simulink model "uz_codegen"  (R2025a)
settings: Solver=FixedStepDiscrete  StartTime=0.0  StopTime=50  RelTol=1e-3  EnableMultiTasking=on
PreLoadFcn:
  | uz_setCodegenPaths
model workspace (MATLAB code in the model file):
  | cmdLim = Simulink.Parameter;
  | cmdLim.Value = 15;
  | cmdLim.Description = 'Limit for controlling the maximum surface command angle.';
  | cmdLim.Min = 0;
  | cmdLim.Max = 90;
  | cmdLim.DocUnits = 'deg';
  | 
  | dispGain = Simulink.Parameter;
  | dispGain.Value = 0.75;
  | dispGain.Description = 'Gain applied to the displacement error.';
  | dispGain.Min = 0;
  | dispGain.Max = [];
  | dispGain.DocUnits = 'deg/sec/deg';
  | 
  | dispLim = Simulink.Parameter;
  | dispLim.Value = 30;
  | dispLim.Description = 'Limit for controlling the maximum commanded angle.';
  | dispLim.Min = 0;
  | dispLim.Max = 180;
  | dispLim.DocUnits = 'deg';
  | 
  | intGain = Simulink.Parameter;
  | intGain.Value = 0.5;
  | intGain.Description = 'Gain applied to the integral error.';
  | intGain.Min = 0;
  | intGain.Max = [];
  | intGain.DocUnits = 'deg/sec/deg/sec';
  | 
  | intLim = Simulink.Parameter;
  | intLim.Value = 5;
  | intLim.Description = 'Limit for controlling the maximum commanded angle.';
  | intLim.Min = 0;
  | intLim.Max = 90;
  | intLim.DocUnits = 'deg';
  | 
  | rateGain = Simulink.Parameter;
  | rateGain.Value = 2;
  | rateGain.Description = 'Gain applied to the rate error.';
  | rateGain.Min = 0;
  | rateGain.Max = [];
  | rateGain.DocUnits = 'deg/deg/sec';
  | 
  | rateLim = Simulink.Parameter;
  | rateLim.Value = 6;
  | rateLim.Description = 'Limit for controlling the maximum commanded angle.';
  | rateLim.Min = 0;
  | rateLim.Max = 180;
  | rateLim.DocUnits = 'deg/sec';
  | 
  | hdgGain = Simulink.Parameter;
  | hdgGain.Value = 0.015;
values from neighbouring files (symbols this model uses):
  DIVIDE_ONE_BY_SQRT_THREE = Simulink.Parameter    [PMSMctrl_param.m]
  GAIN_RADS_TO_HZ = Simulink.Parameter    [PMSMctrl_param.m]
  GAIN_UMIN_TO_HZ = Simulink.Parameter    [PMSMctrl_param.m]
  struct_Ctrl_Config = Simulink.Parameter    [config_Ctrl.m]    (also in paramCtrl.m)
  struct_Inv_Config = Simulink.Parameter    [Inverter_Config.m]
  struct_PMSM_Config = Simulink.Parameter    [PMSM_Config.m]
  struct_ZM_In = Simulink.Parameter    [config_Bus_ZM_in.m]
undefined symbols (not defined in the file or in its folder): ctrl_Tsample, mosfet_deadtime, pwr_Udc, Soll_Regelungsart_en
libraries: mySLLib x8, simulink x7, simulink_extras x2
settings Model: RequirementInfo={} %GIDa_fe9045fd_0412_4b6e_8206_617cc20e6fde  FPTRunName=Active  Creator=ts  LastModifiedBy=jonat
settings SolverCC: AlgebraicLoopSolver=TrustRegion  PositivePriorityOrder=on  AutoInsertRateTranBlk=on
settings DataIOCC: SaveOutput=off  SignalLogging=off  DSMLogging=off  SaveTime=off
settings OptimizationCC: DefaultParameterBehavior=Inlined  UseDivisionForNetSlopeComputation=on  GainParamInheritBuiltInType=on  UseFloatMulNetSlope=on  UseSpecifiedMinMax=on  InlineInvariantSignals=on  PassReuseOutputArgsAs=Individual arguments  NoFixptDivByZeroProtection=on  EfficientFloat2IntCast=on  LifeSpan=1  MaxStackSize=64  OptimizeBlockOrder=speed  DifferentSizesBufferReuse=on  EfficientTunableParamExpr=on
settings DebuggingCC: UnconnectedInputMsg=warning  UnconnectedOutputMsg=warning  UnconnectedLineMsg=warning  BusObjectLabelMismatch=error  AllowSymbolicDim=off  SFUnexpectedBacktrackingDiag=warning  SFNoUnconditionalDefaultTransitionDiag=warning  SFExecutionAtInitializationDiag=none  ArithmeticOperatorsInVariantConditions=warning
settings HardwareCC: ProdBitPerPointer=32.0  ProdBitPerSizeT=32.0  ProdBitPerPtrDiffT=32.0  ProdLargestAtomicInteger=Long  ProdLargestAtomicFloat=Double  ProdWordSize=32.0  ProdLongLongMode=on  ProdHWDeviceType=ARM Compatible->ARM Cortex-R  HardwareBoardFeatureSet=SoCBlockset
settings ModelReferenceCC: EnableRefExpFcnMdlSchedulingChecks=on
settings SFSimCC: MATLABDynamicMemAlloc=off
settings RTWCC: SystemTargetFile=ert.tlc  GenCodeOnly=on  TemplateMakefile=ert_default_tmf  GenerateReport=on  BuildConfiguration=Faster Runs  IncludeHyperlinkInReport=on  DataTypeReplacement=CDataTypesFixedWidth  GenerateCodeMetricsReport=on  CheckMdlBeforeBuild=Warning  GPUComputeCapability=3.5  DLArmComputeVersion=19.05  Description=Embedded Coder
settings CodeAppCC: ForceParamTrailComments=on  IgnoreCustomStorageClasses=off  OperatorAnnotations=on  SimulinkDataObjDesc=on  SFDataObjDesc=on  MATLABFcnDesc=on  CustomSymbolStrGlobalVar=rt$N$M  CustomSymbolStrType=$N$M  CustomSymbolStrFcn=$N$M$F  CustomSymbolStrMacro=$N$M  InsertBlockDesc=on  StateflowObjectComments=on  MATLABSourceComments=on  EnableCustomComments=on  ReqsInCode=on
settings ERTTargetCC: ExtModeTransport=0.0  ExtModeStaticAlloc=off  ExtModeMexFile=ext_comm  ExtModeIntrfLevel=Level1  MultiInstanceErrorCode=Warning  RootIOFormat=Part of model data structure  ERTCustomFileTemplate=example_file_process.tlc  GlobalDataDefinition=InSourceFile  GlobalDataReference=InSourceFile  ERTFilePackagingFormat=CompactWithDataFile  MaxIdInt64=INT64_MAX  MinIdInt64=INT64_MIN  MaxIdUint64=UINT64_MAX  MaxIdInt32=INT32_MAX  MinIdInt32=INT32_MIN  MaxIdUint32=UINT32_MAX  MaxIdInt16=INT16_MAX  MinIdInt16=INT16_MIN  MaxIdUint16=UINT16_MAX  MaxIdInt8=INT8_MAX  MinIdInt8=INT8_MIN  MaxIdUint8=UINT8_MAX  DynamicArrayContainerType=coder::array  TargetLangStandard=C99 (ISO)  CodeReplacementLibrary=GNU C99 extensions  MultiwordLength=2048.0  IncludeMdlTerminateFcn=off  CombineSignalStateStructs=on  SuppressErrorStatus=on  IncludeFileDelimiter=UseQuote  SupportAbsoluteTime=off  CodeInterfacePackaging=Reusable function  SupportNonFinite=off  RemoveResetFunc=off  ParenthesesLevel=Minimum
settings ConfigComp: CovScope=ReferencedModels  CovSaveName=covdata_rollAP  CovMetricSettings=dcmtrwe  CovHTMLOptions=-sRT=1 -aTS=1 -bRG=1 -bTC=1 -hTR=1 -nFC=0 -scm=1 -bcm=1 -xEv=0  CovSaveCumulativeToWorkspaceVar=on  CovSaveSingleToWorkspaceVar=on  CovCumulativeVarName=covCumulativeData_rollAP  CovReportOnPause=off  CovExternalEMLEnable=off  CovSFcnEnable=off

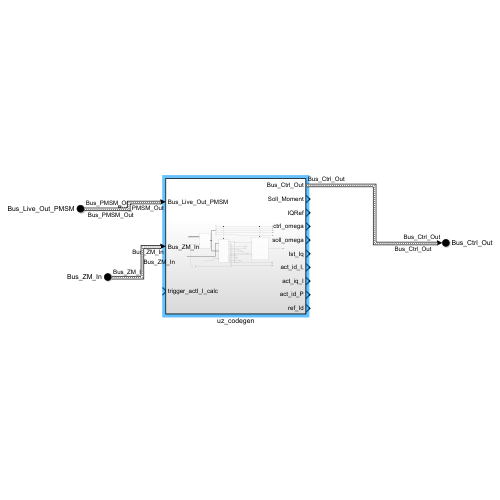
[thumbnail: Simulink's stored preview of the top-level diagram]
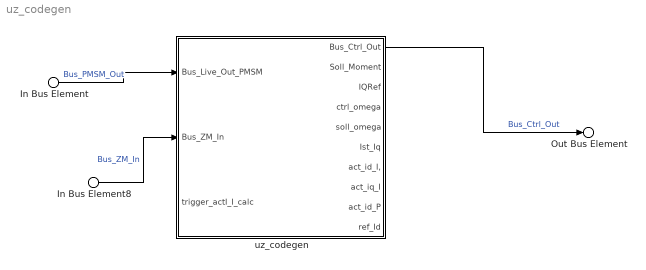
== system uz_codegen ==
  In Bus Element : Inport  PortName=Bus_Live_Out_PMSM
  In Bus Element8 : Inport  Port=2  PortName=Bus_ZM_In
  uz_codegen : Subsystem
  Out Bus Element : Outport  PortName=Bus_Ctrl_Out
  wires:
  In Bus Element8/1 -> uz_codegen/2(Bus_ZM_In)  "Bus_ZM_In"
  In Bus Element/1 -> uz_codegen/1(Bus_Live_Out_PMSM)  "Bus_PMSM_Out"
  uz_codegen/1(Bus_Ctrl_Out) -> Out Bus Element/1  "Bus_Ctrl_Out"

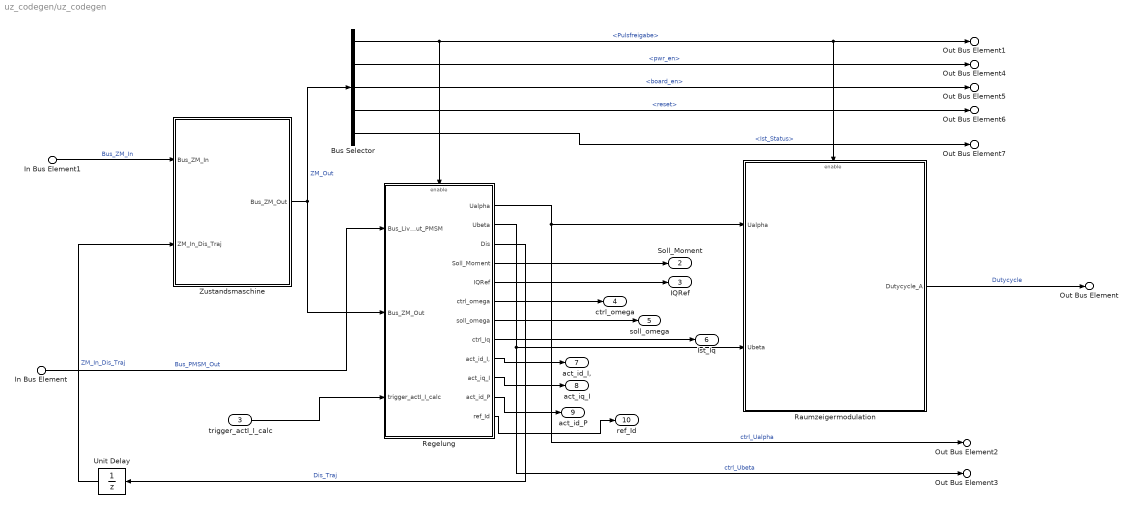
== system uz_codegen/uz_codegen ==
  In Bus Element : Inport  PortName=Bus_Live_Out_PMSM
  In Bus Element1 : Inport  Port=2  PortName=Bus_ZM_In
  trigger_actI_I_calc : Inport  Port=3
  Bus Selector : BusSelector  OutputSignals=Pulsfreigabe,pwr_en,board_en,reset,Ist_Status
  Raumzeigermodulation : Subsystem  TreatAsAtomicUnit=on
      settings: RTWFcnNameOpts=Use subsystem name
  Regelung : Subsystem
      settings: RTWFcnNameOpts=Use subsystem name
  Unit Delay : UnitDelay  SampleTime=-1  HasFrameUpgradeWarning=on
  Zustandsmaschine : Subsystem  TreatAsAtomicUnit=on
      settings: RTWFcnNameOpts=Use subsystem name
  Out Bus Element : Outport  PortName=Bus_Ctrl_Out  Element=Dutycycle
  Out Bus Element1 : Outport  PortName=Bus_Ctrl_Out  Element=act_pwm
  Out Bus Element2 : Outport  PortName=Bus_Ctrl_Out  Element=ctrl_Ualpha_V
  Out Bus Element3 : Outport  PortName=Bus_Ctrl_Out  Element=ctrl_Ubeta_V
  Out Bus Element4 : Outport  PortName=Bus_Ctrl_Out  Element=pwr_en
  Out Bus Element5 : Outport  PortName=Bus_Ctrl_Out  Element=board_en
  Out Bus Element6 : Outport  PortName=Bus_Ctrl_Out  Element=reset
  Out Bus Element7 : Outport  PortName=Bus_Ctrl_Out  Element=ZM_Ist_Status
  Soll_Moment : Outport  Port=2
  IQRef : Outport  Port=3
  ctrl_omega : Outport  Port=4
  soll_omega : Outport  Port=5
  Ist_Iq : Outport  Port=6
  act_id_I, : Outport  Port=7
  act_iq_I : Outport  Port=8
  act_id_P : Outport  Port=9
  ref_Id : Outport  Port=10
  wires:
  Bus Selector/3 -> Out Bus Element5/1  "<board_en>"
  Regelung/3(Dis) -> Unit Delay/1  "Dis_Traj"
  Regelung/1(Ualpha) -> Out Bus Element2/1, Raumzeigermodulation/1(Ualpha)  "ctrl_Ualpha"
  Regelung/2(Ubeta) -> Out Bus Element3/1, Raumzeigermodulation/2(Ubeta)  "ctrl_Ubeta"
  Zustandsmaschine/1(Bus_ZM_Out) -> Regelung/2(Bus_ZM_Out), Bus Selector/1  "ZM_Out"
  Bus Selector/4 -> Out Bus Element6/1  "<reset>"
  Unit Delay/1 -> Zustandsmaschine/2(ZM_In_Dis_Traj)  "ZM_In_Dis_Traj"
  In Bus Element1/1 -> Zustandsmaschine/1(Bus_ZM_In)  "Bus_ZM_In"
  Raumzeigermodulation/1(Dutycycle_A) -> Out Bus Element/1  "Dutycycle"
  Bus Selector/1 -> Regelung/Enable, Raumzeigermodulation/Enable, Out Bus Element1/1  "<Pulsfreigabe>"
  Bus Selector/5 -> Out Bus Element7/1  "<Ist_Status>"
  In Bus Element/1 -> Regelung/1(Bus_Live_Out_PMSM)  "Bus_PMSM_Out"
  Bus Selector/2 -> Out Bus Element4/1  "<pwr_en>"
  Regelung/4(Soll_Moment) -> Soll_Moment/1
  Regelung/5(IQRef) -> IQRef/1
  Regelung/6(ctrl_omega) -> ctrl_omega/1
  Regelung/7(soll_omega) -> soll_omega/1
  Regelung/8(ctrl_Iq) -> Ist_Iq/1
  Regelung/9(act_id_I,) -> act_id_I,/1
  Regelung/10(act_iq_I) -> act_iq_I/1
  Regelung/11(act_id_P) -> act_id_P/1
  Regelung/12(ref_Id) -> ref_Id/1
  trigger_actI_I_calc/1 -> Regelung/3(trigger_actI_I_calc)

== system uz_codegen/uz_codegen/Raumzeigermodulation ==
  Ualpha : Inport
  Ubeta : Inport  Port=2
  Enable : EnablePort
  Constant : Constant  Value=struct_Inv_Config.Udc
  MinimaleSchaltzeit : Subsystem
      settings: RTWFcnNameOpts=Use subsystem name
  Mux : Mux  Inputs=3
  Terminator : Terminator
  Terminator1 : Terminator
  raumzeigermodulation : MATLAB Function  TreatAsAtomicUnit=on
      settings: RTWFcnNameOpts=Use subsystem name
  Dutycycle_A : Outport
  wires:
  MinimaleSchaltzeit/1(Out1) -> Dutycycle_A/1
  Mux/1 -> MinimaleSchaltzeit/1(Dutycycle)
  Ubeta/1 -> raumzeigermodulation/2(Ubeta)  "ctrl_Ubeta"
  Ualpha/1 -> raumzeigermodulation/1(Ualpha)  "ctrl_Ualpha"
  raumzeigermodulation/1(Dutycycle_A) -> Mux/1
  raumzeigermodulation/2(Dutycycle_B) -> Mux/2
  raumzeigermodulation/3(Dutycycle_C) -> Mux/3
  Constant/1 -> raumzeigermodulation/3(Udc)
  raumzeigermodulation/4(Sektor) -> Terminator1/1  "Sektor"
  raumzeigermodulation/5(Quadrant) -> Terminator/1

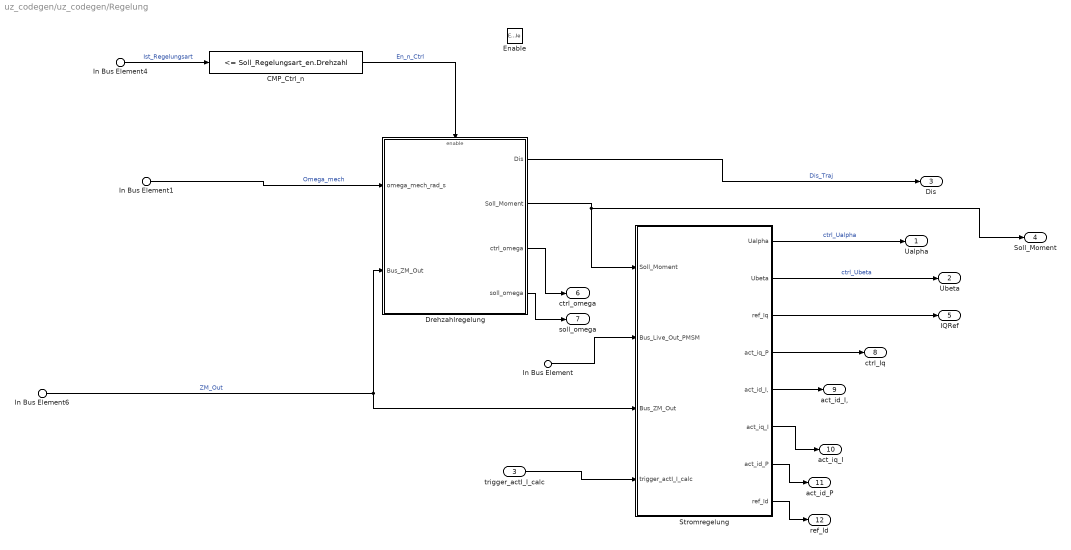
== system uz_codegen/uz_codegen/Regelung ==
  In Bus Element : Inport  PortName=Bus_Live_Out_PMSM
  In Bus Element1 : Inport  PortName=Bus_Live_Out_PMSM  Element=pmsm_Omega_mech_rad_s
  In Bus Element6 : Inport  Port=2  PortName=Bus_ZM_Out
  In Bus Element4 : Inport  Port=2  PortName=Bus_ZM_Out  Element=Ist_Regelungsart
  trigger_actI_I_calc : Inport  Port=3
  Enable : EnablePort  StatesWhenEnabling=reset
  CMP_Ctrl_n : simulink/Logic and Bit Operations/Compare To Constant  relop=<=  const=Soll_Regelungsart_en.Drehzahl  OutDataTypeStr=boolean
  Drehzahlregelung : Subsystem
      settings: RTWFcnNameOpts=Use subsystem name
  Stromregelung : Subsystem  TreatAsAtomicUnit=on
      settings: RTWFcnNameOpts=Use subsystem name
  Ualpha : Outport
  Ubeta : Outport  Port=2
  Dis : Outport  Port=3  OutDataTypeStr=boolean
  Soll_Moment : Outport  Port=4
  IQRef : Outport  Port=5
  ctrl_omega : Outport  Port=6
  soll_omega : Outport  Port=7
  ctrl_Iq : Outport  Port=8
  act_id_I, : Outport  Port=9
  act_iq_I : Outport  Port=10
  act_id_P : Outport  Port=11
  ref_Id : Outport  Port=12
  wires:
  CMP_Ctrl_n/1 -> Drehzahlregelung/Enable  "En_n_Ctrl"
  Drehzahlregelung/2(Soll_Moment) -> Stromregelung/1(Soll_Moment), Soll_Moment/1
  Drehzahlregelung/1(Dis) -> Dis/1  "Dis_Traj"
  In Bus Element1/1 -> Drehzahlregelung/1(omega_mech_rad_s)  "Omega_mech"
  In Bus Element4/1 -> CMP_Ctrl_n/1  "Ist_Regelungsart"
  In Bus Element6/1 -> Drehzahlregelung/2(Bus_ZM_Out), Stromregelung/3(Bus_ZM_Out)  "ZM_Out"
  Stromregelung/2(Ubeta) -> Ubeta/1  "ctrl_Ubeta"
  Stromregelung/1(Ualpha) -> Ualpha/1  "ctrl_Ualpha"
  In Bus Element/1 -> Stromregelung/2(Bus_Live_Out_PMSM)
  Stromregelung/3(ref_Iq) -> IQRef/1
  Drehzahlregelung/3(ctrl_omega) -> ctrl_omega/1
  Drehzahlregelung/4(soll_omega) -> soll_omega/1
  Stromregelung/4(act_iq_P) -> ctrl_Iq/1
  Stromregelung/5(act_id_I,) -> act_id_I,/1
  Stromregelung/6(act_iq_I) -> act_iq_I/1
  Stromregelung/7(act_id_P) -> act_id_P/1
  Stromregelung/8(ref_Id) -> ref_Id/1
  trigger_actI_I_calc/1 -> Stromregelung/4(trigger_actI_I_calc)

== system uz_codegen/uz_codegen/Zustandsmaschine ==
  In Bus Element1 : Inport  PortName=Bus_ZM_In
  ZM_In_Dis_Traj : Inport  Port=2
  state_chart : Stateflow chart  TreatAsAtomicUnit=on
      settings: RTWSystemCode=Nonreusable function  RTWFcnNameOpts=Use subsystem name  FunctionInterfaceSpec=Allow arguments (Optimized)
  Out Bus Element : Outport  PortName=Bus_ZM_Out
  wires:
  ZM_In_Dis_Traj/1 -> state_chart/2(Dis)  "Dis_Traj"
  In Bus Element1/1 -> state_chart/1(Bus_ZM_In)  "Bus_ZM_In"
  state_chart/1(Bus_ZM_Out) -> Out Bus Element/1  "ZM_Out"

== system uz_codegen/uz_codegen/Raumzeigermodulation/MinimaleSchaltzeit ==
  Dutycycle : Inport
  Constant : Constant  Value=struct_Ctrl_Config.IGBT_dc_min
  Constant1 : Constant  Value=0  OutDataTypeStr=single
  Constant2 : Constant  Value=1-struct_Ctrl_Config.IGBT_dc_min
  Constant3 : Constant  OutDataTypeStr=single
  Switch1 : Switch  Threshold=struct_Ctrl_Config.IGBT_dc_min  OutDataTypeStr=single  SaturateOnIntegerOverflow=off  InputSameDT=off
  Switch2 : Switch  Threshold=struct_Ctrl_Config.IGBT_dc_min/2  OutDataTypeStr=single  SaturateOnIntegerOverflow=off  InputSameDT=off
  Switch3 : Switch  Criteria=u2 > Threshold  Threshold=1-struct_Ctrl_Config.IGBT_dc_min  OutDataTypeStr=single  SaturateOnIntegerOverflow=off  InputSameDT=off
  Switch4 : Switch  Threshold=1-struct_Ctrl_Config.IGBT_dc_min/2  OutDataTypeStr=single  SaturateOnIntegerOverflow=off
  Out1 : Outport
  wires:
  Constant/1 -> Switch2/1
  Constant2/1 -> Switch4/3
  Switch3/1 -> Out1/1
  Switch2/1 -> Switch1/3
  Constant3/1 -> Switch4/1
  Dutycycle/1 -> Switch1/2, Switch1/1, Switch2/2
  Switch1/1 -> Switch3/3, Switch3/2, Switch4/2
  Constant1/1 -> Switch2/3
  Switch4/1 -> Switch3/1

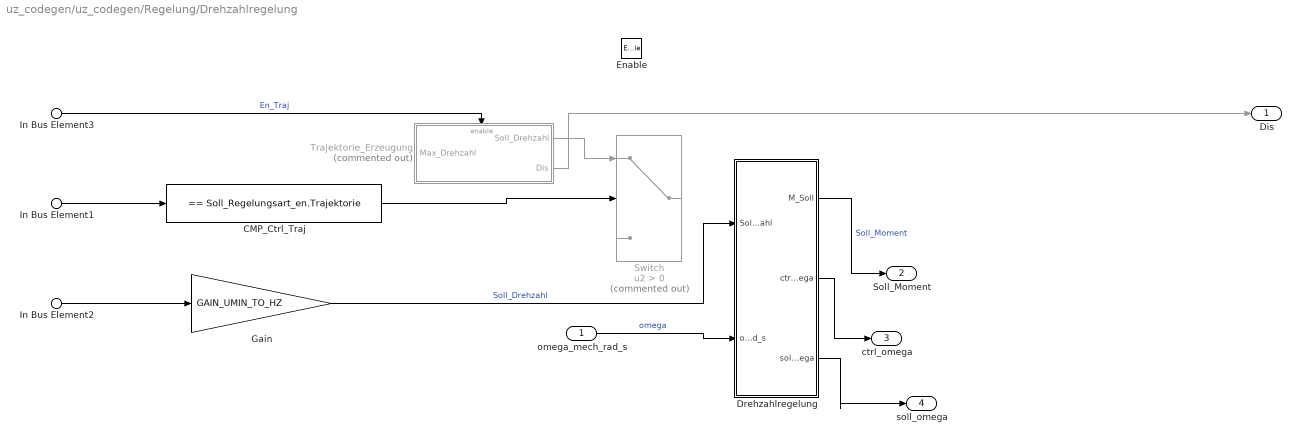
== system uz_codegen/uz_codegen/Regelung/Drehzahlregelung ==
  omega_mech_rad_s : Inport
  In Bus Element3 : Inport  Port=2  PortName=Bus_ZM_Out  Element=En_Traj
  In Bus Element1 : Inport  Port=2  PortName=Bus_ZM_Out  Element=Ist_Regelungsart
  In Bus Element2 : Inport  Port=2  PortName=Bus_ZM_Out  Element=Soll_Drehzahl_Umin
  Enable : EnablePort  StatesWhenEnabling=reset
  CMP_Ctrl_Traj : simulink/Logic and Bit Operations/Compare To Constant  relop===  const=Soll_Regelungsart_en.Trajektorie  OutDataTypeStr=boolean
  Drehzahlregelung : Subsystem
      settings: RTWSystemCode=Nonreusable function  RTWFcnNameOpts=Use subsystem name
  Gain : Gain  Gain=GAIN_UMIN_TO_HZ  RndMeth=Zero
  Switch : Switch  Commented=on  Criteria=u2 > Threshold  SaturateOnIntegerOverflow=off  InputSameDT=off
  Trajektorie_Erzeugung : Subsystem  Commented=on
      settings: RTWSystemCode=Nonreusable function  RTWFcnNameOpts=Use subsystem name
  Dis : Outport
  Soll_Moment : Outport  Port=2
  ctrl_omega : Outport  Port=3
  soll_omega : Outport  Port=4
  wires:
  omega_mech_rad_s/1 -> Drehzahlregelung/2(omega_mech_rad_s)  "omega"
  In Bus Element3/1 -> Trajektorie_Erzeugung/Enable  "En_Traj"
  CMP_Ctrl_Traj/1 -> Switch/2
  In Bus Element1/1 -> CMP_Ctrl_Traj/1
  In Bus Element2/1 -> Gain/1
  Trajektorie_Erzeugung/2(Dis) -> Dis/1
  Gain/1 -> Drehzahlregelung/1(Soll_Drehzahl)  "Soll_Drehzahl"
  Drehzahlregelung/1(M_Soll) -> Soll_Moment/1  "Soll_Moment"
  Trajektorie_Erzeugung/1(Soll_Drehzahl) -> Switch/1
  Drehzahlregelung/2(ctrl_omega) -> ctrl_omega/1
  Drehzahlregelung/3(soll_omega) -> soll_omega/1

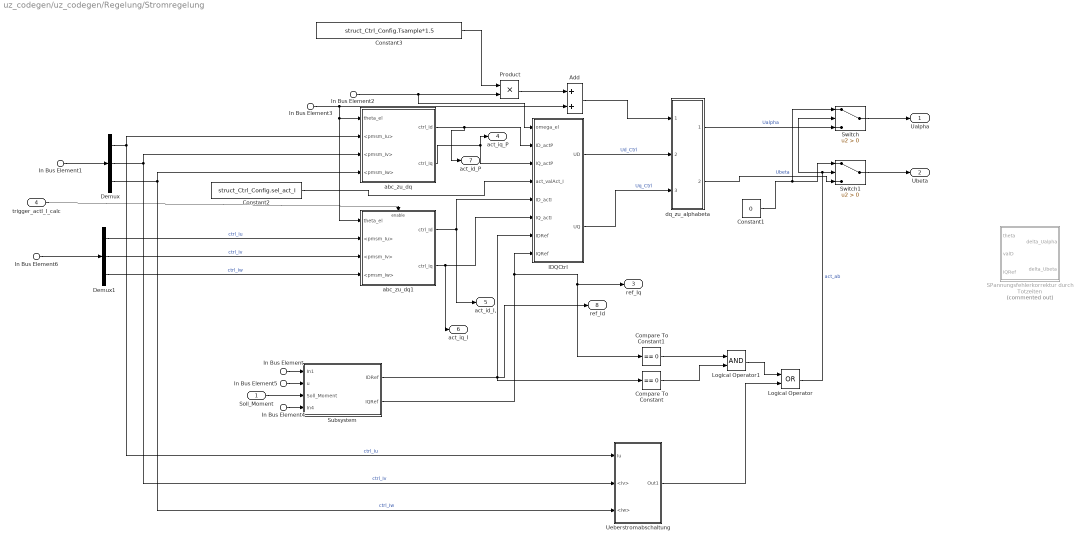
== system uz_codegen/uz_codegen/Regelung/Stromregelung ==
  Soll_Moment : Inport
  In Bus Element1 : Inport  Port=2  PortName=Bus_Live_Out_PMSM  Element=pmsm_Iuvw_P_A
  In Bus Element6 : Inport  Port=2  PortName=Bus_Live_Out_PMSM  Element=pmsm_Iuvw_I_A
  In Bus Element2 : Inport  Port=2  PortName=Bus_Live_Out_PMSM  Element=pmsm_Omega_el_rad_s
  In Bus Element3 : Inport  Port=2  PortName=Bus_Live_Out_PMSM  Element=pmsm_theta_el_rad
  In Bus Element5 : Inport  Port=3  PortName=Bus_ZM_Out  Element=Ist_Regelungsart
  In Bus Element : Inport  Port=3  PortName=Bus_ZM_Out  Element=Soll_id_A
  In Bus Element4 : Inport  Port=3  PortName=Bus_ZM_Out  Element=Soll_iq_A
  trigger_actI_I_calc : Inport  Port=4  OutDataTypeStr=boolean
  Add : Sum
  Compare To Constant : simulink/Logic and Bit Operations/Compare To Constant  relop===  const=0  OutDataTypeStr=boolean
  Compare To Constant1 : simulink/Logic and Bit Operations/Compare To Constant  relop===  const=0  OutDataTypeStr=boolean
  Constant1 : Constant  Value=0  OutDataTypeStr=single
  Constant2 : Constant  Value=struct_Ctrl_Config.sel_act_I  OutDataTypeStr=boolean
  Constant3 : Constant  Value=struct_Ctrl_Config.Tsample*1.5  OutDataTypeStr=single
  Demux : Demux  Outputs=3
  Demux1 : Demux  Outputs=3
  IDQCtrl : Subsystem
      settings: RTWSystemCode=Nonreusable function  RTWFcnNameOpts=Use subsystem name
  Logical Operator : Logic  Operator=OR  AllPortsSameDT=off  OutDataTypeStr=boolean
  Logical Operator1 : Logic  AllPortsSameDT=off  OutDataTypeStr=boolean
  Product : Product
  SPannungsfehlerkorrektur durch Totzeiten : Subsystem  Commented=on
  Subsystem : Subsystem
  Switch : Switch  Criteria=u2 > Threshold  SaturateOnIntegerOverflow=off  InputSameDT=off
  Switch1 : Switch  Criteria=u2 > Threshold  SaturateOnIntegerOverflow=off  InputSameDT=off
  Ueberstromabschaltung : Subsystem
      settings: RTWSystemCode=Nonreusable function  RTWFcnNameOpts=Use subsystem name
  abc_zu_dq : Subsystem
      settings: RTWFcnNameOpts=Use subsystem name
  abc_zu_dq1 : Subsystem
      settings: RTWFcnNameOpts=Use subsystem name
  dq_zu_alphabeta : Subsystem  AncestorBlock=mySLLib/Inverse Park-Transformation
      settings: RTWFcnNameOpts=Use subsystem name
  Ualpha : Outport
  Ubeta : Outport  Port=2
  ref_Iq : Outport  Port=3
  act_iq_P : Outport  Port=4
  act_id_I, : Outport  Port=5
  act_iq_I : Outport  Port=6
  act_id_P : Outport  Port=7
  ref_Id : Outport  Port=8
  wires:
  Logical Operator1/1 -> Logical Operator/1
  Constant3/1 -> Product/1
  In Bus Element1/1 -> Demux/1
  Compare To Constant1/1 -> Logical Operator1/1
  abc_zu_dq/2(ctrl_Iq) -> act_iq_P/1, IDQCtrl/3(IQ_actP)
  abc_zu_dq/1(ctrl_Id) -> act_id_P/1, IDQCtrl/2(ID_actP)
  Compare To Constant/1 -> Logical Operator1/2
  Ueberstromabschaltung/1(Out1) -> Logical Operator/2
  Logical Operator/1 -> Switch/2, Switch1/2  "act_ab"
  Constant1/1 -> Switch/1, Switch1/1
  Switch/1 -> Ualpha/1
  Switch1/1 -> Ubeta/1
  dq_zu_alphabeta/1(valAlpha) -> Switch/3  "Ualpha"
  dq_zu_alphabeta/2(valBeta) -> Switch1/3  "Ubeta"
  IDQCtrl/2(UQ) -> dq_zu_alphabeta/3(valQ)  "Uq_Ctrl"
  Add/1 -> dq_zu_alphabeta/1(theta_el)
  Product/1 -> Add/1
  Demux/1 -> abc_zu_dq/2(<pmsm_Iu>), Ueberstromabschaltung/1(Iu)  "ctrl_Iu"
  Demux/2 -> abc_zu_dq/3(<pmsm_Iv>), Ueberstromabschaltung/2(<Iv>)  "ctrl_Iv"
  In Bus Element3/1 -> abc_zu_dq/1(theta_el), abc_zu_dq1/1(theta_el), Add/2
  Demux/3 -> abc_zu_dq/4(<pmsm_Iw>), Ueberstromabschaltung/3(<Iw>)  "ctrl_Iw"
  In Bus Element2/1 -> IDQCtrl/1(omega_el), Product/2
  IDQCtrl/1(UD) -> dq_zu_alphabeta/2(valD)  "Ud_Ctrl"
  Constant2/1 -> IDQCtrl/4(act_valAct_I)
  Subsystem/1(IDRef) -> ref_Id/1, IDQCtrl/7(IDRef), Compare To Constant/1
  Subsystem/2(IQRef) -> IDQCtrl/8(IQRef), Compare To Constant1/1, ref_Iq/1
  In Bus Element/1 -> Subsystem/1(In1)
  In Bus Element5/1 -> Subsystem/2(u)
  Soll_Moment/1 -> Subsystem/3(Soll_Moment)
  In Bus Element4/1 -> Subsystem/4(In4)
  abc_zu_dq1/1(ctrl_Id) -> IDQCtrl/5(ID_actI), act_id_I,/1
  abc_zu_dq1/2(ctrl_Iq) -> act_iq_I/1, IDQCtrl/6(IQ_actI)
  Demux1/1 -> abc_zu_dq1/2(<pmsm_Iu>)  "ctrl_Iu"
  Demux1/2 -> abc_zu_dq1/3(<pmsm_Iv>)  "ctrl_Iv"
  Demux1/3 -> abc_zu_dq1/4(<pmsm_Iw>)  "ctrl_Iw"
  In Bus Element6/1 -> Demux1/1
  trigger_actI_I_calc/1 -> abc_zu_dq1/Enable

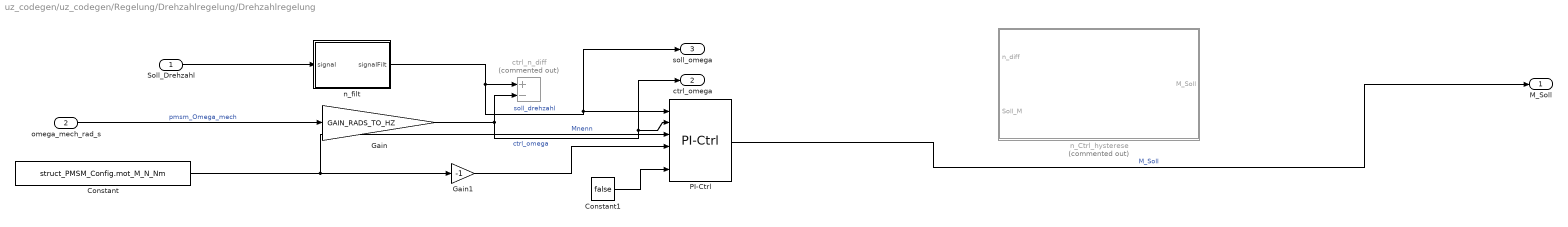
== system uz_codegen/uz_codegen/Regelung/Drehzahlregelung/Drehzahlregelung ==
  Soll_Drehzahl : Inport  OutDataTypeStr=single
  omega_mech_rad_s : Inport  Port=2
  Constant : Constant  Value=struct_PMSM_Config.mot_M_N_Nm  SampleTime=-1
  Constant1 : Constant  Value=false  OutDataTypeStr=boolean
  Gain : Gain  Gain=GAIN_RADS_TO_HZ  OutDataTypeStr=single  RndMeth=Zero
  Gain1 : Gain  Gain=-1
  PI-Ctrl : mySLLib/PI-Ctrl  localGain=struct_Ctrl_Config.KPn  localTsample=struct_Ctrl_Config.Tsample  localKi=struct_Ctrl_Config.KIn
      settings: SourceProductName=MSSS Bibliothek
  ctrl_n_diff : Sum  Commented=on  Inputs=+-
  n_Ctrl_hysterese : Subsystem  Commented=on  TreatAsAtomicUnit=on
  n_filt : Subsystem  AncestorBlock=libKollege/low pass filter  mask{localTFilt=struct_Ctrl_Config.TNn, localTsample=struct_Ctrl_Config.Tsample}
      mask prompts: localTFilt "Filterzeitkonstante (s)"; localTsample "Abtastzeit (s)"
      mask init:
      | if localTsample <= 0
      |     error('Abtastzeit darf nicht kleiner gleich Null sein!')
      | end
      | 
      | if localTFilt <= 0
      |     error('Filterzeit darf nicht kleiner gleich Null sein!')
      | end
  M_Soll : Outport  OutDataTypeStr=single
  ctrl_omega : Outport  Port=2
  soll_omega : Outport  Port=3
  wires:
  Gain1/1 -> PI-Ctrl/4
  Soll_Drehzahl/1 -> n_filt/1(signal)
  omega_mech_rad_s/1 -> Gain/1  "pmsm_Omega_mech"
  Constant/1 -> Gain1/1, PI-Ctrl/3  "Mnenn"
  Gain/1 -> ctrl_omega/1, PI-Ctrl/2, ctrl_n_diff/2  "ctrl_omega"
  n_filt/1(signalFilt) -> ctrl_n_diff/1, soll_omega/1, PI-Ctrl/1  "soll_drehzahl"
  PI-Ctrl/1 -> M_Soll/1  "M_Soll"
  Constant1/1 -> PI-Ctrl/6

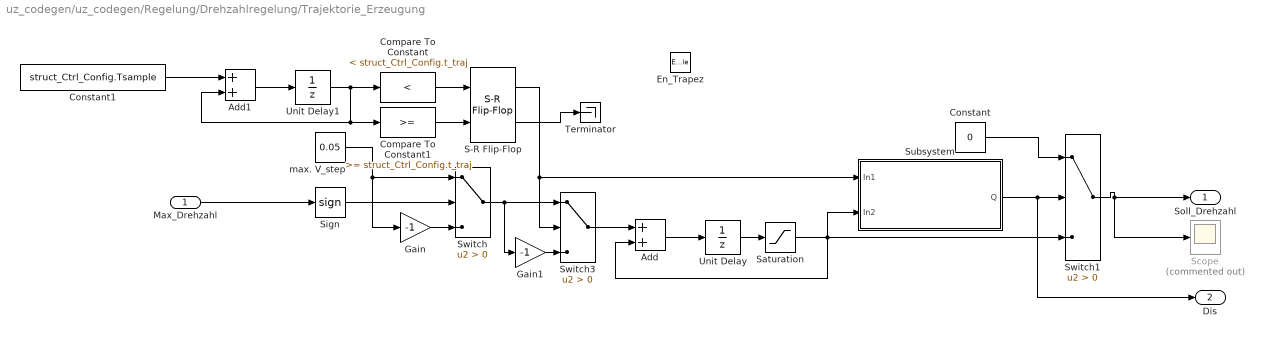
== system uz_codegen/uz_codegen/Regelung/Drehzahlregelung/Trajektorie_Erzeugung ==
  Max_Drehzahl : Inport  OutDataTypeStr=single
  En_Trapez : EnablePort  StatesWhenEnabling=reset
  Add : Sum  OutDataTypeStr=single
  Add1 : Sum  OutDataTypeStr=single
  Compare To Constant : simulink/Logic and Bit Operations/Compare To Constant  relop=<  const=struct_Ctrl_Config.t_traj  OutDataTypeStr=boolean
  Compare To Constant1 : simulink/Logic and Bit Operations/Compare To Constant  relop=>=  const=struct_Ctrl_Config.t_traj  OutDataTypeStr=boolean
  Constant : Constant  Value=0  OutDataTypeStr=single
  Constant1 : Constant  Value=struct_Ctrl_Config.Tsample
  Gain : Gain  Gain=-1
  Gain1 : Gain  Gain=-1
  S-R Flip-Flop : simulink_extras/Flip Flops/S-R Flip-Flop  initial_condition=1
  Saturation : Saturate  UpperLimit=abs(struct_ZM_In.Soll_Drehzahl)  LowerLimit=-abs(struct_ZM_In.Soll_Drehzahl)
  Scope : Scope  Commented=on
      settings: ActiveDisplayYMinimum=-9.860748565205089  ActiveDisplayYMaximum=4.6148882593554967
  Sign : Signum
  Subsystem : Subsystem  TreatAsAtomicUnit=on
      settings: RTWSystemCode=Inline
  Switch : Switch  Criteria=u2 > Threshold  OutDataTypeStr=single  SaturateOnIntegerOverflow=off  InputSameDT=off
  Switch1 : Switch  Criteria=u2 > Threshold  OutDataTypeStr=single  SaturateOnIntegerOverflow=off  InputSameDT=off
  Switch3 : Switch  Criteria=u2 > Threshold  OutDataTypeStr=single  SaturateOnIntegerOverflow=off  InputSameDT=off
  Terminator : Terminator
  Unit Delay : UnitDelay  SampleTime=-1  HasFrameUpgradeWarning=on
  Unit Delay1 : UnitDelay  SampleTime=-1  HasFrameUpgradeWarning=on
  max. V_step : Constant  Value=0.05  OutDataTypeStr=single  LockScale=on
  Soll_Drehzahl : Outport  OutDataTypeStr=single
  Dis : Outport  Port=2
  wires:
  S-R Flip-Flop/2 -> Terminator/1
  Subsystem/1(Q) -> Switch1/2, Dis/1
  Constant/1 -> Switch1/1
  Switch1/1 -> Soll_Drehzahl/1, Scope/1
  Saturation/1 -> Add/2, Switch1/3, Subsystem/2(In2)
  Compare To Constant1/1 -> S-R Flip-Flop/2
  Unit Delay1/1 -> Compare To Constant1/1, Add1/2, Compare To Constant/1
  Compare To Constant/1 -> S-R Flip-Flop/1
  S-R Flip-Flop/1 -> Subsystem/1(In1), Switch3/2
  Gain1/1 -> Switch3/3
  Switch3/1 -> Add/1
  Constant1/1 -> Add1/1
  Add1/1 -> Unit Delay1/1
  Sign/1 -> Switch/2
  Gain/1 -> Switch/3
  max. V_step/1 -> Switch/1, Gain/1
  Switch/1 -> Switch3/1, Gain1/1
  Unit Delay/1 -> Saturation/1
  Add/1 -> Unit Delay/1
  Max_Drehzahl/1 -> Sign/1

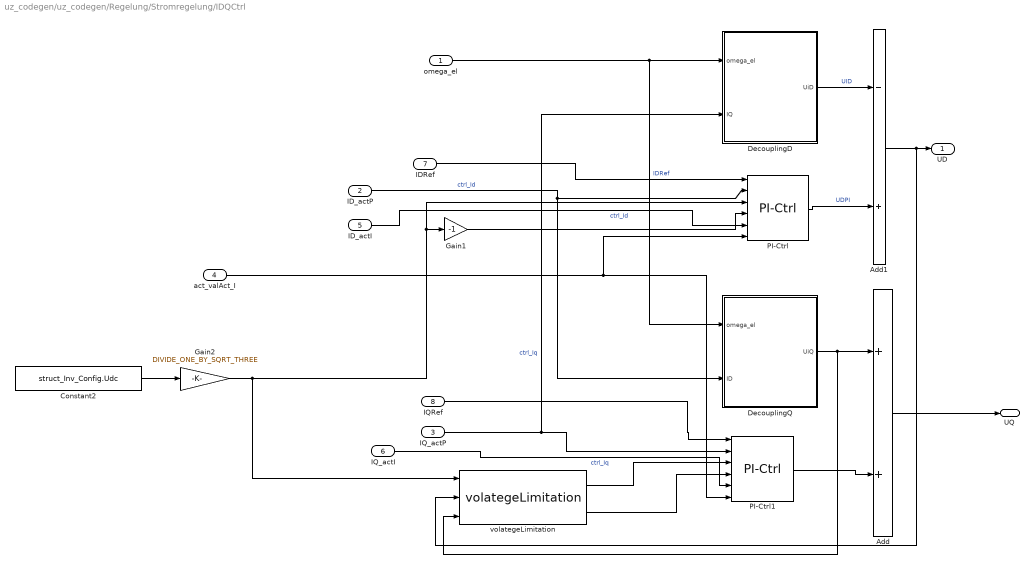
== system uz_codegen/uz_codegen/Regelung/Stromregelung/IDQCtrl ==
  omega_el : Inport
  ID_actP : Inport  Port=2
  IQ_actP : Inport  Port=3
  act_valAct_I : Inport  Port=4
  ID_actI : Inport  Port=5
  IQ_actI : Inport  Port=6
  IDRef : Inport  Port=7
  IQRef : Inport  Port=8
  Add : Sum
  Add1 : Sum  Inputs=-+
  Constant2 : Constant  Value=struct_Inv_Config.Udc  SampleTime=-1
  DecouplingD : Subsystem
  DecouplingQ : Subsystem
  Gain1 : Gain  Gain=-1
  Gain2 : Gain  Gain=DIVIDE_ONE_BY_SQRT_THREE
  PI-Ctrl : mySLLib/PI-Ctrl  localGain=struct_Ctrl_Config.KPi  localTsample=struct_Ctrl_Config.Tsample  localKi=struct_Ctrl_Config.KIi
      settings: SourceProductName=MSSS Bibliothek
  PI-Ctrl1 : mySLLib/PI-Ctrl  localGain=struct_Ctrl_Config.KPi  localTsample=struct_Ctrl_Config.Tsample  localKi=struct_Ctrl_Config.KIi
      settings: SourceProductName=MSSS Bibliothek
  volategeLimitation : mySLLib/volategeLimitation
      settings: SourceProductName=MSSS Bibliothek
  UD : Outport
  UQ : Outport  Port=2
  wires:
  volategeLimitation/2 -> PI-Ctrl1/4
  volategeLimitation/1 -> PI-Ctrl1/3
  ID_actP/1 -> DecouplingQ/2(ID), PI-Ctrl/2  "ctrl_Id"
  Add/1 -> UQ/1
  Gain1/1 -> PI-Ctrl/4
  Gain2/1 -> volategeLimitation/1, PI-Ctrl/3, Gain1/1
  DecouplingQ/1(UiQ) -> Add/1, volategeLimitation/3
  Add1/1 -> UD/1, volategeLimitation/2
  DecouplingD/1(UiD) -> Add1/1  "UID"
  PI-Ctrl/1 -> Add1/2  "UDPI"
  omega_el/1 -> DecouplingD/1(omega_el), DecouplingQ/1(omega_el)
  PI-Ctrl1/1 -> Add/2
  IQ_actP/1 -> DecouplingD/2(IQ), PI-Ctrl1/2  "ctrl_Iq"
  IDRef/1 -> PI-Ctrl/1  "IDRef"
  IQRef/1 -> PI-Ctrl1/1
  Constant2/1 -> Gain2/1
  ID_actI/1 -> PI-Ctrl/5  "ctrl_Id"
  act_valAct_I/1 -> PI-Ctrl1/6, PI-Ctrl/6
  IQ_actI/1 -> PI-Ctrl1/5  "ctrl_Iq"

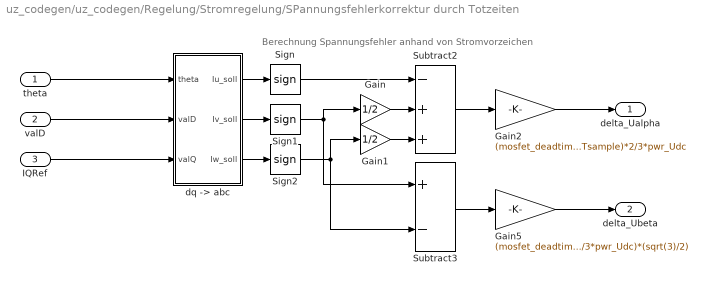
== system uz_codegen/uz_codegen/Regelung/Stromregelung/SPannungsfehlerkorrektur durch Totzeiten ==
  note: Berechnung Spannungsfehler anhand von Stromvorzeichen
  theta : Inport
  valD : Inport  Port=2
  IQRef : Inport  Port=3
  Gain : Gain  Gain=1/2
  Gain1 : Gain  Gain=1/2
  Gain2 : Gain  Gain=(mosfet_deadtime/ctrl_Tsample)*2/3*pwr_Udc
  Gain5 : Gain  Gain=(mosfet_deadtime/ctrl_Tsample)*(2/3*pwr_Udc)*(sqrt(3)/2)
  Sign : Signum
  Sign1 : Signum
  Sign2 : Signum
  Subtract2 : Sum  Inputs=-++
  Subtract3 : Sum  Inputs=+-
  "dq -> abc" : Subsystem
  delta_Ualpha : Outport
  delta_Ubeta : Outport  Port=2
  wires:
  Gain2/1 -> delta_Ualpha/1
  theta/1 -> "dq -> abc"/1(theta)
  Gain5/1 -> delta_Ubeta/1
  IQRef/1 -> "dq -> abc"/3(valQ)
  valD/1 -> "dq -> abc"/2(valD)
  "dq -> abc"/2(Iv_soll) -> Sign1/1
  "dq -> abc"/3(Iw_soll) -> Sign2/1
  Gain1/1 -> Subtract2/3
  "dq -> abc"/1(Iu_soll) -> Sign/1
  Subtract3/1 -> Gain5/1
  Sign2/1 -> Gain1/1, Subtract3/2
  Gain/1 -> Subtract2/2
  Sign1/1 -> Gain/1, Subtract3/1
  Subtract2/1 -> Gain2/1
  Sign/1 -> Subtract2/1

== system uz_codegen/uz_codegen/Regelung/Stromregelung/Subsystem ==
  In1 : Inport
  u : Inport  Port=2
  Soll_Moment : Inport  Port=3
  In4 : Inport  Port=4
  Compare To Constant2 : simulink/Logic and Bit Operations/Compare To Constant  relop===  const=Soll_Regelungsart_en.Strom  OutDataTypeStr=boolean
  Constant : Constant  Value=0  OutDataTypeStr=single
  Switch2 : Switch  Criteria=u2 > Threshold  SaturateOnIntegerOverflow=off  InputSameDT=off
  Switch3 : Switch  Criteria=u2 > Threshold  SaturateOnIntegerOverflow=off  InputSameDT=off
  calcIq : Subsystem  TreatAsAtomicUnit=on
      settings: RTWSystemCode=Inline
  IDRef : Outport
  IQRef : Outport  Port=2
  wires:
  Soll_Moment/1 -> calcIq/1(M)
  Compare To Constant2/1 -> Switch2/2, Switch3/2
  In4/1 -> Switch3/1
  Constant/1 -> Switch2/3
  Switch2/1 -> IDRef/1  "IDRef"
  calcIq/1(Iq) -> Switch3/3
  u/1 -> Compare To Constant2/1
  Switch3/1 -> IQRef/1  "IQRef"
  In1/1 -> Switch2/1

== system uz_codegen/uz_codegen/Regelung/Stromregelung/Ueberstromabschaltung ==
  Iu : Inport
  <Iv> : Inport  Port=2
  <Iw> : Inport  Port=3
  Abs : Abs  SaturateOnIntegerOverflow=off
  Abs1 : Abs  SaturateOnIntegerOverflow=off
  Abs2 : Abs  SaturateOnIntegerOverflow=off
  Constant : Constant  Value=struct_PMSM_Config.mot_I_max_A
  Logical Operator : Logic  Operator=OR  Inputs=3  AllPortsSameDT=off  OutDataTypeStr=boolean
  Relational Operator : RelationalOperator  Operator=<  OutDataTypeStr=boolean  RndMeth=Simplest  InputSameDT=off
  Relational Operator1 : RelationalOperator  Operator=<  OutDataTypeStr=boolean  RndMeth=Simplest  InputSameDT=off
  Relational Operator2 : RelationalOperator  Operator=<  OutDataTypeStr=boolean  RndMeth=Simplest  InputSameDT=off
  Out1 : Outport
  wires:
  Constant/1 -> Relational Operator/1, Relational Operator1/1, Relational Operator2/1
  Relational Operator2/1 -> Logical Operator/3
  Relational Operator1/1 -> Logical Operator/2
  Relational Operator/1 -> Logical Operator/1
  Logical Operator/1 -> Out1/1
  Abs2/1 -> Relational Operator2/2
  Abs1/1 -> Relational Operator1/2
  Abs/1 -> Relational Operator/2
  <Iw>/1 -> Abs2/1
  <Iv>/1 -> Abs1/1
  Iu/1 -> Abs/1

== system uz_codegen/uz_codegen/Regelung/Stromregelung/abc_zu_dq ==
  theta_el : Inport
  <pmsm_Iu> : Inport  Port=2
  <pmsm_Iv> : Inport  Port=3
  <pmsm_Iw> : Inport  Port=4
  Clarke-Transformation : mySLLib/Clarke-Transformation  SystemSampleTime=-1  VariantActivationTime=update diagram  EmptyChoice=off  PassThrough=off  PassThroughVariantControl=(default)  EmptyChoiceVariantControl=(default)  AllowFlexibleInterface=on  Latency=0  AutoFrameSizeCalculation=off
      link override Gain: Gain=DIVIDE_TWO_BY_THREE
      link override Gain1: Gain=DIVIDE_TWO_BY_THREE
      link override Gain5: Gain=DIVIDE_SQRT_THREE_BY_TWO
      link override sqrt(3)//2: Gain=-DIVIDE_SQRT_THREE_BY_TWO
      settings: SourceProductName=MSSS Bibliothek
  Park-Transformation : Subsystem  AncestorBlock=mySLLib/Park-Transformation
  ctrl_Id : Outport
  ctrl_Iq : Outport  Port=2
  wires:
  <pmsm_Iw>/1 -> Clarke-Transformation/3
  theta_el/1 -> Park-Transformation/1(theta)
  <pmsm_Iv>/1 -> Clarke-Transformation/2
  Park-Transformation/2(valQ) -> ctrl_Iq/1  "ctrl_Iq"
  <pmsm_Iu>/1 -> Clarke-Transformation/1
  Clarke-Transformation/1 -> Park-Transformation/2(valAlpha)
  Park-Transformation/1(valD) -> ctrl_Id/1  "ctrl_Id"
  Clarke-Transformation/2 -> Park-Transformation/3(valBeta)

== system uz_codegen/uz_codegen/Regelung/Stromregelung/abc_zu_dq1 ==
  theta_el : Inport
  <pmsm_Iu> : Inport  Port=2
  <pmsm_Iv> : Inport  Port=3
  <pmsm_Iw> : Inport  Port=4
  Enable : EnablePort
  Clarke-Transformation : mySLLib/Clarke-Transformation  SystemSampleTime=-1  VariantActivationTime=update diagram  EmptyChoice=off  PassThrough=off  PassThroughVariantControl=(default)  EmptyChoiceVariantControl=(default)  AllowFlexibleInterface=on  Latency=0  AutoFrameSizeCalculation=off
      link override Gain: Gain=DIVIDE_TWO_BY_THREE
      link override Gain1: Gain=DIVIDE_TWO_BY_THREE
      link override Gain5: Gain=DIVIDE_SQRT_THREE_BY_TWO
      link override sqrt(3)//2: Gain=-DIVIDE_SQRT_THREE_BY_TWO
      settings: SourceProductName=MSSS Bibliothek
  Park-Transformation : Subsystem  AncestorBlock=mySLLib/Park-Transformation
  ctrl_Id : Outport
  ctrl_Iq : Outport  Port=2
  wires:
  Clarke-Transformation/2 -> Park-Transformation/3(valBeta)
  Park-Transformation/1(valD) -> ctrl_Id/1  "ctrl_Id"
  Clarke-Transformation/1 -> Park-Transformation/2(valAlpha)
  <pmsm_Iu>/1 -> Clarke-Transformation/1
  Park-Transformation/2(valQ) -> ctrl_Iq/1  "ctrl_Iq"
  <pmsm_Iv>/1 -> Clarke-Transformation/2
  theta_el/1 -> Park-Transformation/1(theta)
  <pmsm_Iw>/1 -> Clarke-Transformation/3

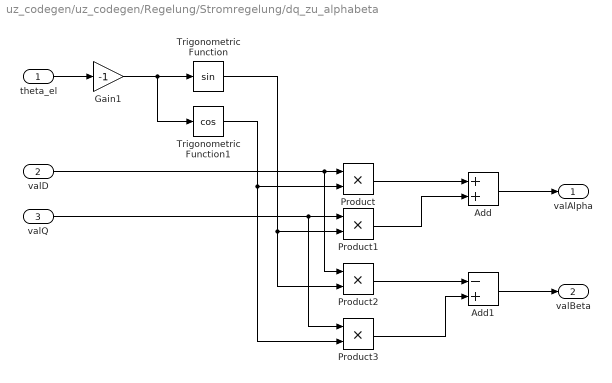
== system uz_codegen/uz_codegen/Regelung/Stromregelung/dq_zu_alphabeta ==
  theta_el : Inport
  valD : Inport  Port=2
  valQ : Inport  Port=3
  Add : Sum
  Add1 : Sum  Inputs=-+
  Gain1 : Gain  Gain=-1
  Product{,1..3} (4 alike) : Product
  Trigonometric Function : Trigonometry  OutputSignalType=real
  Trigonometric Function1 : Trigonometry  Operator=cos  OutputSignalType=real
  valAlpha : Outport
  valBeta : Outport  Port=2
  wires:
  theta_el/1 -> Gain1/1
  Add/1 -> valAlpha/1
  Add1/1 -> valBeta/1
  Gain1/1 -> Trigonometric Function1/1, Trigonometric Function/1
  valD/1 -> Product2/1, Product/1
  Trigonometric Function1/1 -> Product3/2, Product/2
  valQ/1 -> Product1/1, Product3/1
  Product/1 -> Add/1
  Product1/1 -> Add/2
  Trigonometric Function/1 -> Product2/2, Product1/2
  Product2/1 -> Add1/1
  Product3/1 -> Add1/2

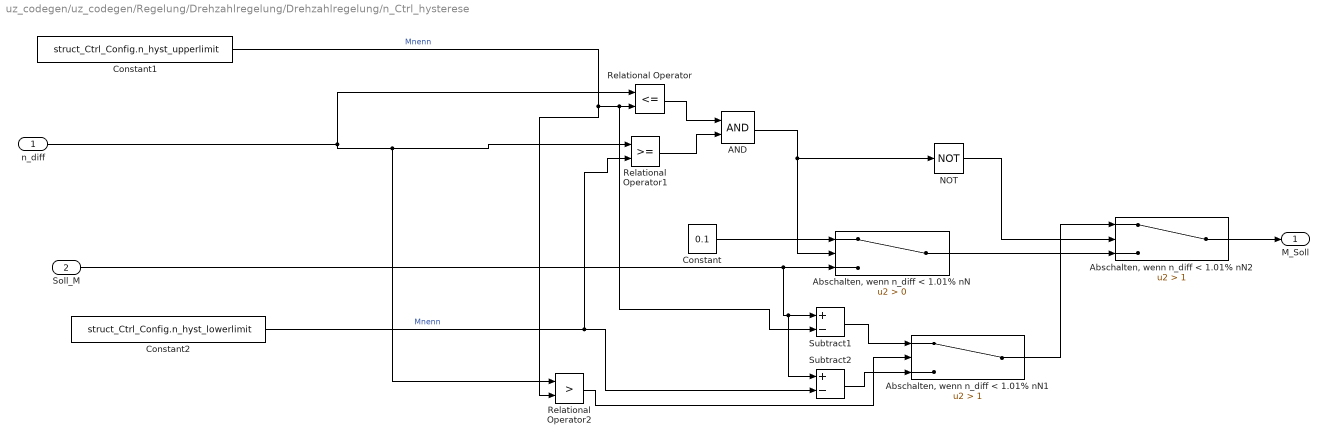
== system uz_codegen/uz_codegen/Regelung/Drehzahlregelung/Drehzahlregelung/n_Ctrl_hysterese ==
  n_diff : Inport
  Soll_M : Inport  Port=2
  AND : Logic  AllPortsSameDT=off  OutDataTypeStr=boolean
  "Abschalten, wenn n_diff < 1.01% nN" : Switch  Criteria=u2 > Threshold  SaturateOnIntegerOverflow=off  InputSameDT=off
  "Abschalten, wenn n_diff < 1.01% nN1" : Switch  Criteria=u2 > Threshold  Threshold=1  SaturateOnIntegerOverflow=off  InputSameDT=off
  "Abschalten, wenn n_diff < 1.01% nN2" : Switch  Criteria=u2 > Threshold  Threshold=1  SaturateOnIntegerOverflow=off  InputSameDT=off
  Constant : Constant  Value=0.1  OutDataTypeStr=single
  Constant1 : Constant  Value=struct_Ctrl_Config.n_hyst_upperlimit
  Constant2 : Constant  Value=struct_Ctrl_Config.n_hyst_lowerlimit
  NOT : Logic  Operator=NOT  IconShape=distinctive  AllPortsSameDT=off  OutDataTypeStr=boolean
  Relational Operator : RelationalOperator  Operator=<=  OutDataTypeStr=boolean  RndMeth=Simplest  InputSameDT=off
  Relational Operator1 : RelationalOperator  OutDataTypeStr=boolean  RndMeth=Simplest  InputSameDT=off
  Relational Operator2 : RelationalOperator  Operator=>  OutDataTypeStr=boolean  RndMeth=Simplest  InputSameDT=off
  Subtract1 : Sum  Inputs=+-
  Subtract2 : Sum  Inputs=+-
  M_Soll : Outport
  wires:
  Constant1/1 -> Relational Operator/2, Subtract1/2, Relational Operator2/2  "Mnenn"
  "Abschalten, wenn n_diff < 1.01% nN1"/1 -> "Abschalten, wenn n_diff < 1.01% nN2"/1
  n_diff/1 -> Relational Operator1/1, Relational Operator2/1, Relational Operator/1
  Relational Operator1/1 -> AND/2
  Constant2/1 -> Subtract2/2, Relational Operator1/2  "Mnenn"
  Relational Operator2/1 -> "Abschalten, wenn n_diff < 1.01% nN1"/2
  NOT/1 -> "Abschalten, wenn n_diff < 1.01% nN2"/2
  AND/1 -> "Abschalten, wenn n_diff < 1.01% nN"/2, NOT/1
  Subtract2/1 -> "Abschalten, wenn n_diff < 1.01% nN1"/3
  Relational Operator/1 -> AND/1
  Subtract1/1 -> "Abschalten, wenn n_diff < 1.01% nN1"/1
  "Abschalten, wenn n_diff < 1.01% nN"/1 -> "Abschalten, wenn n_diff < 1.01% nN2"/3
  Constant/1 -> "Abschalten, wenn n_diff < 1.01% nN"/1
  Soll_M/1 -> "Abschalten, wenn n_diff < 1.01% nN"/3, Subtract1/1, Subtract2/1
  "Abschalten, wenn n_diff < 1.01% nN2"/1 -> M_Soll/1

== system uz_codegen/uz_codegen/Regelung/Drehzahlregelung/Drehzahlregelung/n_filt ==
  note: Integrator
  signal : Inport
  Add : Sum
  Add1 : Sum  Inputs=+-
  Constant3 : Constant  Value=localTsample/localTFilt
  Product2 : Product
  Unit Delay : UnitDelay  SampleTime=-1  HasFrameUpgradeWarning=on
  signalFilt : Outport
  wires:
  Constant3/1 -> Product2/1
  Add/1 -> Unit Delay/1
  Product2/1 -> Add/1
  Add1/1 -> Product2/2
  Unit Delay/1 -> Add1/2, signalFilt/1, Add/2
  signal/1 -> Add1/1

== system uz_codegen/uz_codegen/Regelung/Drehzahlregelung/Trajektorie_Erzeugung/Subsystem ==
  In1 : Inport
  In2 : Inport  Port=2  OutDataTypeStr=single
  Relational Operator : RelationalOperator  Operator=~=  OutDataTypeStr=boolean  RndMeth=Simplest  InputSameDT=off
  S-R Flip-Flop1 : simulink_extras/Flip Flops/S-R Flip-Flop  initial_condition=0
  Scope : Scope  NumInputPorts=2
      settings: ActiveDisplayYMinimum=-1.25  ActiveDisplayYMaximum=1.25
  Sign1 : Signum
  Terminator : Terminator
  Unit Delay2 : UnitDelay  InitialCondition=sign(struct_ZM_In.Soll_Drehzahl)  SampleTime=-1  HasFrameUpgradeWarning=on
  Q : Outport
  wires:
  S-R Flip-Flop1/2 -> Terminator/1
  In1/1 -> S-R Flip-Flop1/2
  Unit Delay2/1 -> Relational Operator/1, Scope/1
  Sign1/1 -> Unit Delay2/1, Scope/2, Relational Operator/2
  In2/1 -> Sign1/1
  Relational Operator/1 -> S-R Flip-Flop1/1
  S-R Flip-Flop1/1 -> Q/1

== system uz_codegen/uz_codegen/Regelung/Stromregelung/IDQCtrl/DecouplingD ==
  omega_el : Inport
  IQ : Inport  Port=2
  Constant : Constant  Value=struct_PMSM_Config.mot_Lq_H
  Product : Product
  Product1 : Product
  UiD : Outport
  wires:
  Constant/1 -> Product1/2
  Product1/1 -> UiD/1
  Product/1 -> Product1/1
  IQ/1 -> Product/2
  omega_el/1 -> Product/1

== system uz_codegen/uz_codegen/Regelung/Stromregelung/IDQCtrl/DecouplingQ ==
  omega_el : Inport
  ID : Inport  Port=2
  Add : Sum
  Constant : Constant  Value=struct_PMSM_Config.mot_Ld_H  SampleTime=-1
  Constant1 : Constant  Value=struct_PMSM_Config.mot_psi_pm_Vs  SampleTime=-1
  Product : Product
  Product1 : Product
  UiQ : Outport
  wires:
  Constant/1 -> Product1/2
  Constant1/1 -> Add/2
  Add/1 -> Product/2
  Product1/1 -> Add/1
  ID/1 -> Product1/1
  Product/1 -> UiQ/1
  omega_el/1 -> Product/1

== system uz_codegen/uz_codegen/Regelung/Stromregelung/SPannungsfehlerkorrektur durch Totzeiten/dq -> abc ==
  theta : Inport
  valD : Inport  Port=2
  valQ : Inport  Port=3
  Inverse Clarke-Transformation : mySLLib/Inverse Clarke-Transformation  SystemSampleTime=-1  VariantActivationTime=update diagram  EmptyChoice=off  PassThrough=off  PassThroughVariantControl=(default)  EmptyChoiceVariantControl=(default)  AllowFlexibleInterface=on  Latency=0  AutoFrameSizeCalculation=off
      settings: SourceProductName=MSSS Bibliothek
  Inverse Park-Transformation1 : mySLLib/Inverse Park-Transformation  SystemSampleTime=-1  VariantActivationTime=update diagram  EmptyChoice=off  PassThrough=off  PassThroughVariantControl=(default)  EmptyChoiceVariantControl=(default)  AllowFlexibleInterface=on  Latency=0  AutoFrameSizeCalculation=off
      settings: SourceProductName=MSSS Bibliothek
  calcRelRefVoltage : Subsystem  Commented=on
  Iu_soll : Outport
  Iv_soll : Outport  Port=2
  Iw_soll : Outport  Port=3
  wires:
  Inverse Clarke-Transformation/2 -> Iv_soll/1  "uV"
  Inverse Clarke-Transformation/3 -> Iw_soll/1  "uW"
  valQ/1 -> Inverse Park-Transformation1/3
  Inverse Clarke-Transformation/1 -> Iu_soll/1  "uU"
  theta/1 -> Inverse Park-Transformation1/1
  Inverse Park-Transformation1/2 -> Inverse Clarke-Transformation/2
  Inverse Park-Transformation1/1 -> Inverse Clarke-Transformation/1
  valD/1 -> Inverse Park-Transformation1/2

== system uz_codegen/uz_codegen/Regelung/Stromregelung/Subsystem/calcIq ==
  M : Inport
  Gain : Gain  Gain=(2/3)/struct_PMSM_Config.mot_psi_pm_Vs/struct_PMSM_Config.mot_p  OutDataTypeStr=single
  Iq : Outport  OutDataTypeStr=single
  wires:
  Gain/1 -> Iq/1
  M/1 -> Gain/1

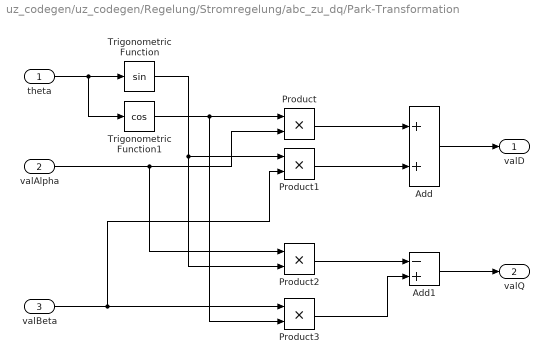
== system uz_codegen/uz_codegen/Regelung/Stromregelung/abc_zu_dq/Park-Transformation ==
  theta : Inport
  valAlpha : Inport  Port=2
  valBeta : Inport  Port=3
  Add : Sum
  Add1 : Sum  Inputs=-+
  Product{,1..3} (4 alike) : Product
  Trigonometric Function : Trigonometry  OutputSignalType=real
  Trigonometric Function1 : Trigonometry  Operator=cos  OutputSignalType=real
  valD : Outport
  valQ : Outport  Port=2
  wires:
  Add1/1 -> valQ/1
  Add/1 -> valD/1
  theta/1 -> Trigonometric Function/1, Trigonometric Function1/1
  valAlpha/1 -> Product2/1, Product/2
  Trigonometric Function1/1 -> Product/1, Product3/2
  valBeta/1 -> Product3/1, Product1/2
  Product1/1 -> Add/2
  Product/1 -> Add/1
  Trigonometric Function/1 -> Product1/1, Product2/2
  Product2/1 -> Add1/1
  Product3/1 -> Add1/2

== system uz_codegen/uz_codegen/Regelung/Stromregelung/abc_zu_dq1/Park-Transformation ==
  theta : Inport
  valAlpha : Inport  Port=2
  valBeta : Inport  Port=3
  Add : Sum
  Add1 : Sum  Inputs=-+
  Product{,1..3} (4 alike) : Product
  Trigonometric Function : Trigonometry  OutputSignalType=real
  Trigonometric Function1 : Trigonometry  Operator=cos  OutputSignalType=real
  valD : Outport
  valQ : Outport  Port=2
  wires:
  Product3/1 -> Add1/2
  Product2/1 -> Add1/1
  Trigonometric Function/1 -> Product2/2, Product1/1
  Product/1 -> Add/1
  Product1/1 -> Add/2
  valBeta/1 -> Product1/2, Product3/1
  Trigonometric Function1/1 -> Product3/2, Product/1
  valAlpha/1 -> Product/2, Product2/1
  theta/1 -> Trigonometric Function1/1, Trigonometric Function/1
  Add/1 -> valD/1
  Add1/1 -> valQ/1

== system uz_codegen/uz_codegen/Regelung/Stromregelung/SPannungsfehlerkorrektur durch Totzeiten/dq -> abc/calcRelRefVoltage ==
  UU : Inport
  UV : Inport  Port=2
  UW : Inport  Port=3
  Udc : Inport  Port=4
  Divide : Product  Inputs=*/
  Divide1 : Product  Inputs=*/
  Divide2 : Product  Inputs=*/
  uU : Outport
  uV : Outport  Port=2
  uW : Outport  Port=3
  wires:
  Udc/1 -> Divide/2, Divide1/2, Divide2/2
  Divide/1 -> uU/1
  Divide1/1 -> uV/1
  Divide2/1 -> uW/1
  UW/1 -> Divide2/1
  UV/1 -> Divide1/1
  UU/1 -> Divide/1

== matlab function uz_codegen/Raumzeigermodulation/raumzeigermodulation ==
  data: Dutycycle_A output single; Dutycycle_B output single; Dutycycle_C output single; Ualpha input single; Ubeta input single; Sektor output single; Quadrant output single; Udc input single
function [Dutycycle_A, Dutycycle_B, Dutycycle_C,  Sektor, Quadrant] = Dutycycle(Ualpha, Ubeta, Udc)
DIVIDE_ONE_BY_SQRT_THREE = single(single(1) / sqrt(3));
DIVIDE_ONE_BY_TWO_THIRDS = single(single(1) / (2/3));
DIVIDE_TWO_BY_TWO_THIRDS = single(2 / (2/3));
Sektor = single(0);
Quadrant = single(0);
Dutycycle_A = single(0);
Dutycycle_B = single(0);
Dutycycle_C = single(0);

abs_Ualpha = abs(Ualpha);
abs_Ubeta = abs(Ubeta);

% Parameter a,b und c berechnen
a = single(((abs_Ualpha + abs_Ubeta*DIVIDE_ONE_BY_SQRT_THREE)*DIVIDE_ONE_BY_TWO_THIRDS)/Udc);
b = single(((abs_Ualpha - abs_Ubeta*DIVIDE_ONE_BY_SQRT_THREE)*DIVIDE_ONE_BY_TWO_THIRDS)/Udc);
c = single((abs_Ubeta*DIVIDE_ONE_BY_SQRT_THREE*DIVIDE_TWO_BY_TWO_THIRDS)/Udc);

% Sektor bestimmen
if Ubeta < 0
	if Ualpha < 0.0
		Quadrant = single(3);
		if b < 0
			Sektor = single(5);
		else
			Sektor = single(4);
        end
	else
		Quadrant = single(4);
		if b < 0
			Sektor = single(5);
		else
			Sektor = single(6);
        end
    end
else
	if Ualpha < 0
		Quadrant = single(2);
		if b < 0
			Sektor = single(2);
		else
        	Sektor = single(3);
        end
	else
		Quadrant = single(1);
		if b < 0
			Sektor = single(2);
		else
			Sektor = single(1);
        end
    end
end

%Dutycycle berechnen
	switch Sektor

    	case single(1)
    		Dutycycle_A = (single(1) + b + c);
    		Dutycycle_B = (single(1) - b + c);
    		Dutycycle_C = (single(1) - b - c);
        
        case 2
            if Quadrant == single(1)
                Dutycycle_A = (single(1) + a + b);
                Dutycycle_B = (single(1) + a - b);
                Dutycycle_C = (single(1) - a + b);
            else
                Dutycycle_A = (single(1) - a - b);
                Dutycycle_B = (single(1) + a - b);
                Dutycycle_C = (single(1) - a + b);
            end

        case 3
            Dutycycle_A = (single(1) - b - c);
            Dutycycle_B = (single(1) + b + c);
            Dutycycle_C = (single(1) + b - c);

        case 4
            Dutycycle_A = (single(1) - b - c);
            Dutycycle_B = (single(1) + b - c);
            Dutycycle_C = (single(1) + b + c);

        case 5
            if Quadrant == 3
                Dutycycle_A = (single(1) - a - b);
                Dutycycle_B = (single(1) - a + b);
                Dutycycle_C = (single(1) + a - b);
            else
                Dutycycle_A = (single(1) + b + a);
                Dutycycle_B = (single(1) + b - a);
                Dutycycle_C = (single(1) - b + a);
            end

        case 6
            Dutycycle_A = (single(1) + b + c);
            Dutycycle_B = (single(1) - b - c);
            Dutycycle_C = (single(1) - b + c);

    end

Dutycycle_A =  Dutycycle_A * single(0.5);
Dutycycle_B =  Dutycycle_B * single(0.5);
Dutycycle_C =  Dutycycle_C * single(0.5);

== stateflow chart uz_codegen/Zustandsmaschine/state_chart ==
  state NoError
    state Idle
      during:
      Bus_ZM_Out.Ist_Status = Status_Ctrl.Ready;
      Bus_ZM_Out.Pulsfreigabe = false;
      Bus_ZM_Out.Ist_Regelungsart = Soll_Regelungsart_en.Drehzahl;
      Bus_ZM_Out.En_Traj=false;
      Bus_ZM_Out.Soll_Drehzahl_Umin = 0;
      Bus_ZM_Out.Soll_id_A = 0;
      Bus_ZM_Out.Soll_iq_A = 0;
      Bus_ZM_Out.reset  = false;
      Bus_ZM_Out.pwr_en  = false;
      Bus_ZM_Out.board_en  = false;
    state Run
      during:
      Bus_ZM_Out.Ist_Status = Status_Ctrl.Run;
      Bus_ZM_Out.Pulsfreigabe = true;
      Bus_ZM_Out.reset  = false;
      Bus_ZM_Out.pwr_en  = true;
      Bus_ZM_Out.board_en  = true;
      state nCtrl
        during:
        Bus_ZM_Out.Ist_Regelungsart = Soll_Regelungsart_en.Drehzahl;
        Bus_ZM_Out.Soll_Drehzahl_Umin = Bus_ZM_In.Soll_Drehzahl_Umin;
        Bus_ZM_Out.Soll_id_A = 0;
        Bus_ZM_Out.Soll_iq_A = 0;
      state Stromregelung
        during:
        Bus_ZM_Out.Soll_id_A = Bus_ZM_In.Soll_id_A;
        Bus_ZM_Out.Soll_iq_A = Bus_ZM_In.Soll_iq_A;
        Bus_ZM_Out.Soll_Drehzahl_Umin = 0;
        Bus_ZM_Out.Ist_Regelungsart = Soll_Regelungsart_en.Strom;
      state Trapez [commented out]
        during:
        Bus_ZM_Out.Ist_Regelungsart = Soll_Regelungsart_en.Trajektorie;
        Bus_ZM_Out.Soll_Drehzahl_Umin = Bus_ZM_In.Soll_Drehzahl_Umin;
        Bus_ZM_Out.Soll_id_A = 0;
        Bus_ZM_Out.Soll_iq_A = 0;
        state Warten [commented out]
          Bus_ZM_Out.En_Traj = false;
        state Run [commented out]
          Bus_ZM_Out.En_Traj = true;
        (default) -> Warten [commented out]
        NoError.Run.Trapez.Run -> Warten [commented out] : [Dis == 1]
        Warten -> NoError.Run.Trapez.Run [commented out] : [Bus_ZM_In.Start_Traj == 1]
      (default) -> nCtrl
      nCtrl -> Stromregelung : [Bus_ZM_In.Soll_Regelungsart == Soll_Regelungsart_en.Strom]
      Stromregelung -> nCtrl : [Bus_ZM_In.Soll_Regelungsart ~= Soll_Regelungsart_en.Strom]
      Trapez -> nCtrl [commented out] : [Dis == 1 || Bus_ZM_In.Soll_Regelungsart ~= Soll_Regelungsart_en.Trajektorie]
      nCtrl -> Trapez [commented out] : [Bus_ZM_In.Soll_Regelungsart == Soll_Regelungsart_en.Trajektorie]
    state Ready
      during:
      Bus_ZM_Out.Ist_Status = Status_Ctrl.Ready;
      Bus_ZM_Out.Pulsfreigabe = false;
      Bus_ZM_Out.Ist_Regelungsart = Soll_Regelungsart_en.Drehzahl;
      Bus_ZM_Out.En_Traj=false;
      Bus_ZM_Out.Soll_Drehzahl_Umin = 0;
      Bus_ZM_Out.Soll_id_A = 0;
      Bus_ZM_Out.Soll_iq_A = 0;
      Bus_ZM_Out.reset  = false;
      Bus_ZM_Out.pwr_en  = true;
      Bus_ZM_Out.board_en  = true;
    (default) -> Idle
    NoError.Run -> Idle : [Bus_ZM_In.UZ_Platform_State == platform_state_t.idle_state || Bus_ZM_In.Inv_Ready == false]
    Ready -> Idle [order 2] : [Bus_ZM_In.UZ_Platform_State == platform_state_t.idle_state]
    Idle -> Ready : [Bus_ZM_In.UZ_Platform_State == platform_state_t.running_state]
    Ready -> NoError.Run [order 1] : [Bus_ZM_In.UZ_Platform_State == platform_state_t.control_state && Bus_ZM_In.Inv_Ready == true]
  state Error
    during:
    Bus_ZM_Out.Ist_Status = Status_Ctrl.Error_Status;
    Bus_ZM_Out.Pulsfreigabe = false;
    Bus_ZM_Out.Ist_Regelungsart = Soll_Regelungsart_en.Error;
    Bus_ZM_Out.En_Traj = false;
    Bus_ZM_Out.Soll_Drehzahl_Umin = 0;
    Bus_ZM_Out.Soll_id_A = 0;
    Bus_ZM_Out.Soll_iq_A = 0;
    Bus_ZM_Out.reset  = true;
    Bus_ZM_Out.pwr_en  = false;
    Bus_ZM_Out.board_en  = false;
  (default) -> NoError
  NoError -> Error : [Bus_ZM_In.Fehlermeldung == true || Bus_ZM_In.UZ_Platform_State == platform_state_t.error_state || Bus_ZM_In.IGBT_desat == true]
  Error -> NoError : [Bus_ZM_In.Fehlermeldung == false && Bus_ZM_In.UZ_Platform_State == platform_state_t.idle_state]
  data: Bus_ZM_In input; Dis input boolean; Bus_ZM_Out output Bus: Bus_ZM_Out
